simulink model "pfd3"  (R2024b)
settings: Solver=FixedStepAuto  StartTime=0.0  StopTime=10.0  FixedStep=Ts  RelTol=1e-3
values from neighbouring files (symbols this model uses):
  bf = t/2    (= 0.6)    [main_data_vehicle.m]
  br = t/2    (= 0.6)    [main_data_vehicle.m]
  lf = L*fr    (= 0.8635)    [main_data_vehicle.m]
  lr = L-lf    (= 0.7065)    [main_data_vehicle.m]
settings Model: Creator=marti  LastModifiedBy=marti

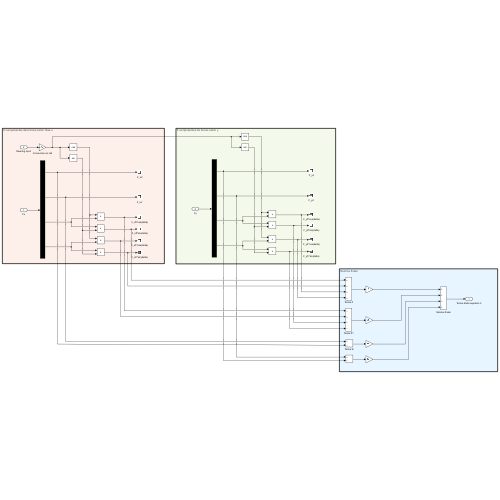
[thumbnail: Simulink's stored preview of the top-level diagram]
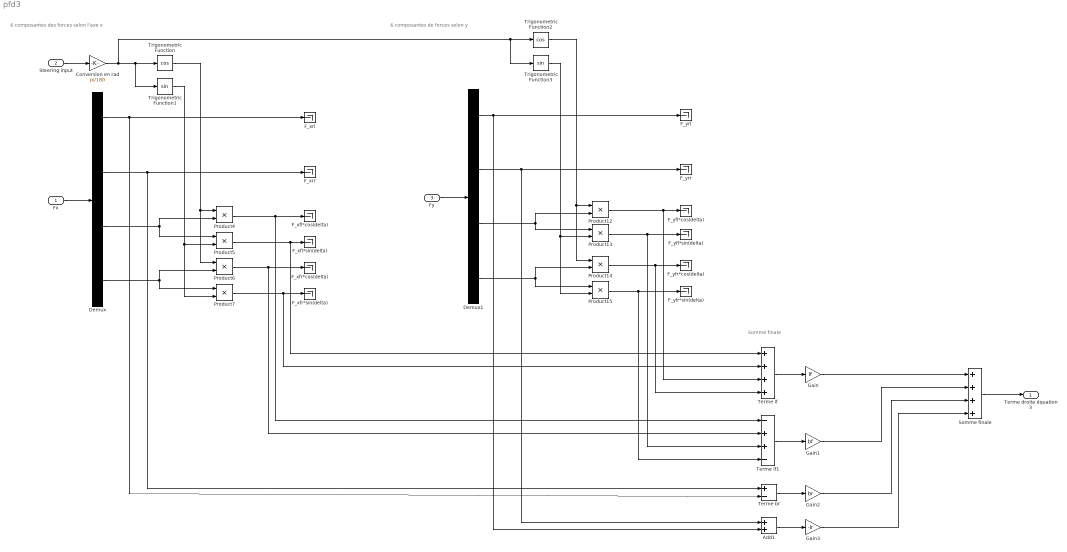
== system pfd3 ==
  note: Somme finale
  note: 6 composantes de forces selon y
  note: 6 composantes des forces selon l'axe x
  Fx : Inport
  Steering input : Inport  Port=2
  Fy : Inport  Port=3
  Add1 : Sum
  Conversion en rad : Gain  Gain=pi/180
  Demux : Demux
  Demux1 : Demux
  F_xfl*cos(delta) : Terminator
  F_xfl*sin(delta) : Terminator
  F_xfr*cos(delta) : Terminator
  F_xfr*sin(delta) : Terminator
  F_xrl : Terminator
  F_xrr : Terminator
  F_yfl*cos(delta) : Terminator
  F_yfl*sin(delta) : Terminator
  F_yfr*cos(delta) : Terminator
  F_yfr*sin(delta) : Terminator
  F_yrl : Terminator
  F_yrr : Terminator
  Gain : Gain  Gain=lf
  Gain1 : Gain  Gain=bf
  Gain2 : Gain  Gain=br
  Gain3 : Gain  Gain=-lr
  Product{4..7,12..15} (8 alike) : Product
  Somme finale : Sum  Inputs=++++
  Terme br : Sum  Inputs=+-
  Terme lf : Sum  Inputs=++++
  Terme lf1 : Sum  Inputs=-++-
  Trigonometric Function : Trigonometry  Operator=cos
  Trigonometric Function1 : Trigonometry
  Trigonometric Function2 : Trigonometry  Operator=cos
  Trigonometric Function3 : Trigonometry
  Terme droite équation 3 : Outport
  wires:
  Fx/1 -> Demux/1
  Conversion en rad/1 -> Trigonometric Function3/1, Trigonometric Function2/1, Trigonometric Function1/1, Trigonometric Function/1
  Terme lf/1 -> Gain/1
  Trigonometric Function/1 -> Product6/1, Product4/1
  Trigonometric Function1/1 -> Product7/2, Product5/2
  Demux/1 -> Terme br/2, F_xrl/1
  Product4/1 -> F_xfl*cos(delta)/1, Terme lf1/1
  Product5/1 -> F_xfl*sin(delta)/1, Terme lf/1
  Demux/3 -> Product5/1, Product4/2
  Product6/1 -> F_xfr*cos(delta)/1, Terme lf1/2
  Product7/1 -> F_xfr*sin(delta)/1, Terme lf/2
  Demux/4 -> Product7/1, Product6/2
  Terme lf1/1 -> Gain1/1
  Demux1/4 -> Product14/2, Product15/1
  Product12/1 -> Terme lf/3, F_yfl*cos(delta)/1
  Steering input/1 -> Conversion en rad/1
  Demux1/1 -> Add1/2, F_yrl/1
  Trigonometric Function3/1 -> Product15/2, Product13/2
  Product14/1 -> Terme lf/4, F_yfr*cos(delta)/1
  Trigonometric Function2/1 -> Product14/1, Product12/1
  Product15/1 -> Terme lf1/4, F_yfr*sin(delta)/1
  Demux1/3 -> Product12/2, Product13/1
  Fy/1 -> Demux1/1
  Product13/1 -> Terme lf1/3, F_yfl*sin(delta)/1
  Demux1/2 -> Add1/1, F_yrr/1
  Terme br/1 -> Gain2/1
  Add1/1 -> Gain3/1
  Demux/2 -> Terme br/1, F_xrr/1
  Gain/1 -> Somme finale/1
  Gain1/1 -> Somme finale/2
  Gain2/1 -> Somme finale/3
  Gain3/1 -> Somme finale/4
  Somme finale/1 -> Terme droite équation 3/1
